simulink model "npsauv_with_psi_converter"  (R2017a)
settings: Solver=FixedStepAuto  StartTime=0.0  StopTime=1000  FixedStep=1  RelTol=1e-3
libraries: simulink x1
settings Model: Creator=admin  LastModifiedBy=WangZhe

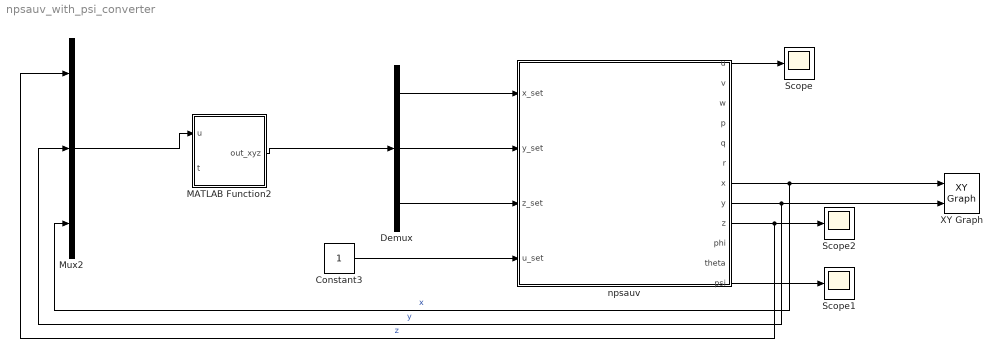
== system npsauv_with_psi_converter ==
  Constant3 : Constant
  Demux : Demux  Outputs=3
  MATLAB Function2 : MATLAB Function  TreatAsAtomicUnit=on
  Mux2 : Mux  Inputs=3
  Scope : Scope
  Scope1 : Scope
  Scope2 : Scope
  XY Graph : simulink/Sinks/XY Graph  xmin=0  xmax=200  ymin=-100  ymax=200  st=-1
  npsauv : Subsystem  mask{x_init=[0.1 0 0 0 0 0 0 0 0 0 0 0]}
      mask prompts: x_init "initial states: [u v w p q r x y z phi theta psi]"
  wires:
  npsauv/8(y) -> Mux2/2, XY Graph/2  "y"
  npsauv/1(u) -> Scope/1
  npsauv/7(x) -> Mux2/3, XY Graph/1  "x"
  npsauv/12(psi) -> Scope1/1
  Constant3/1 -> npsauv/4(u_set)
  Mux2/1 -> MATLAB Function2/1(u)
  Demux/1 -> npsauv/1(x_set)
  Demux/2 -> npsauv/2(y_set)
  MATLAB Function2/1(out_xyz) -> Demux/1
  Demux/3 -> npsauv/3(z_set)
  npsauv/9(z) -> Mux2/1, Scope2/1  "z"

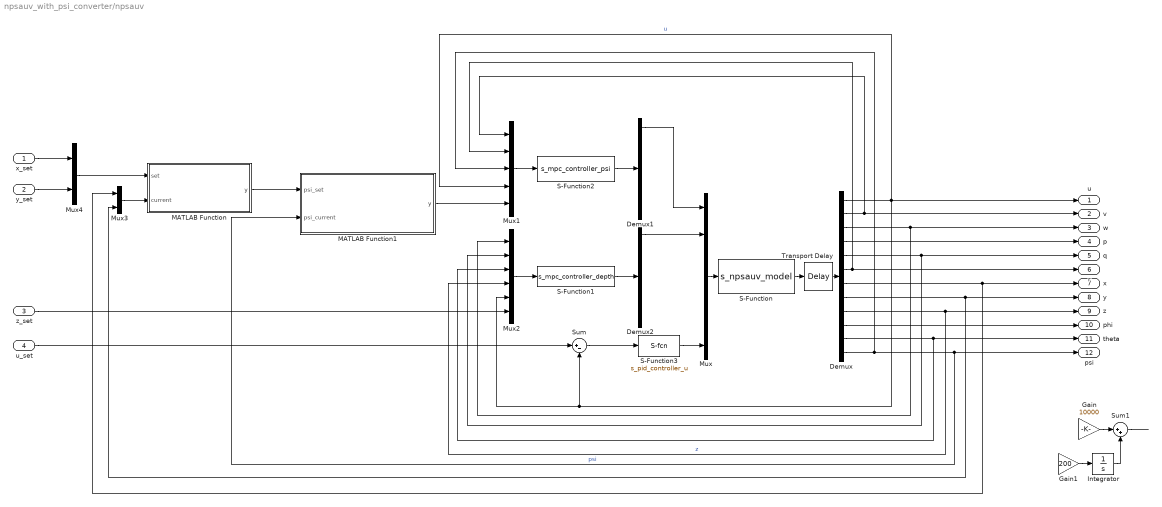
== system npsauv_with_psi_converter/npsauv ==
  x_set : Inport
  y_set : Inport  Port=2
  z_set : Inport  Port=3
  u_set : Inport  Port=4
  Demux : Demux  Outputs=12
  Demux1 : Demux  Outputs=5
  Demux2 : Demux  Outputs=5
  Gain : Gain  Gain=10000
  Gain1 : Gain  Gain=200
  Integrator : Integrator  LimitOutput=on  UpperSaturationLimit=50  LowerSaturationLimit=-50
  MATLAB Function : MATLAB Function  TreatAsAtomicUnit=on
  MATLAB Function1 : MATLAB Function  TreatAsAtomicUnit=on
  Mux : Mux  Inputs=6
  Mux1 : Mux  Inputs=5
  Mux2 : Mux  Inputs=6
  Mux3 : Mux  Inputs=2
  Mux4 : Mux  Inputs=2
  S-Function : S-Function  FunctionName=s_npsauv_model  Parameters=x_init  SFunctionDeploymentMode=off  EnableBusSupport=off
  S-Function1 : S-Function  FunctionName=s_mpc_controller_depth  SFunctionDeploymentMode=off  EnableBusSupport=off
  S-Function2 : S-Function  FunctionName=s_mpc_controller_psi  SFunctionDeploymentMode=off  EnableBusSupport=off
  S-Function3 : S-Function  FunctionName=s_pid_controller_u  SFunctionDeploymentMode=off  EnableBusSupport=off
  Sum : Sum  Inputs=|+-
  Sum1 : Sum  Inputs=|++
  Transport Delay : TransportDelay  DelayTime=0.01
  u : Outport
  v : Outport  Port=2
  w : Outport  Port=3
  p : Outport  Port=4
  q : Outport  Port=5
  r : Outport  Port=6
  x : Outport  Port=7
  y : Outport  Port=8
  z : Outport  Port=9
  phi : Outport  Port=10
  theta : Outport  Port=11
  psi : Outport  Port=12
  wires:
  Demux/9 -> z/1, Mux2/4  "z"
  Mux/1 -> S-Function/1
  Demux2/1 -> Mux/2
  Demux/5 -> Mux2/2, q/1
  z_set/1 -> Mux2/6
  Demux/11 -> theta/1, Mux2/3
  Mux2/1 -> S-Function1/1
  S-Function1/1 -> Demux2/1
  Demux/6 -> r/1, Mux1/2
  Demux/1 -> u/1, Mux2/5, Sum/2, Mux1/4  "u"
  u_set/1 -> Sum/1
  Demux/12 -> MATLAB Function1/2(psi_current), psi/1, Mux1/3  "psi"
  Mux1/1 -> S-Function2/1
  Demux/2 -> Mux1/1, v/1
  Demux1/1 -> Mux/1
  Demux/3 -> Mux2/1, w/1
  S-Function2/1 -> Demux1/1
  MATLAB Function1/1(y) -> Mux1/5
  Demux/4 -> p/1
  Demux/10 -> phi/1
  Integrator/1 -> Sum1/2
  Gain1/1 -> Integrator/1
  Sum1/1 -> ?
  ? -> Gain1/1, Gain/1
  Gain/1 -> Sum1/1
  S-Function3/1 -> Mux/6
  Sum/1 -> S-Function3/1
  S-Function/1 -> Transport Delay/1
  Transport Delay/1 -> Demux/1
  MATLAB Function/1(y) -> MATLAB Function1/1(psi_set)
  Demux/8 -> y/1, Mux3/2
  Mux3/1 -> MATLAB Function/2(current)
  Demux/7 -> x/1, Mux3/1
  Mux4/1 -> MATLAB Function/1(set)
  y_set/1 -> Mux4/2
  x_set/1 -> Mux4/1

== matlab function npsauv_with_psi_converter/npsauv/MATLAB Function1 ==
  data: psi_set input; y output; psi_current input
function y = psi_set_converter(psi_set,psi_current)
%find nearest psi
while psi_set-psi_current>2*pi
    psi_set=psi_set-2*pi;
end
while psi_set-psi_current<=2*pi
    psi_set=psi_set+2*pi;
end
if psi_set-psi_current>pi
    psi_set=psi_set-2*pi;
end
if psi_set-psi_current<-pi
    psi_set=psi_set+2*pi;
end
y=psi_set;

== matlab function npsauv_with_psi_converter/npsauv/MATLAB Function ==
  data: set input; y output; current input
function y = coordinate_to_psi(set,current)
vec=set-current;
y=atan2(vec(2),vec(1));

== matlab function npsauv_with_psi_converter/MATLAB Function2 ==
  data: out_xyz output; u input; t input
function out_xyz = f(u,t)
S = load('pathdata.mat','a');
out_xyz = [1,S.a(1,1),S.a(1,2)*200];
i =2;

while i<22 && tmod
    if  out_xyz(1)-u(1)<0.1 && out_xyz(2)-u(2)<0.1 && out_xyz(3)-u(3)<10
        out_xyz = [1,S.a(i,1),S.a(i,2)*200];
        i =i+1;
    end      
end
